simulink library "rotorTemp_lib"  (R2022b)
settings: Solver=VariableStepAuto  StartTime=0.0  StopTime=10.0  RelTol=1e-3
undefined symbols (not defined in the file): raptor_xcp_function
libraries: Raptor_lib x9
settings Model: Creator=serga  LastModifiedBy=serga

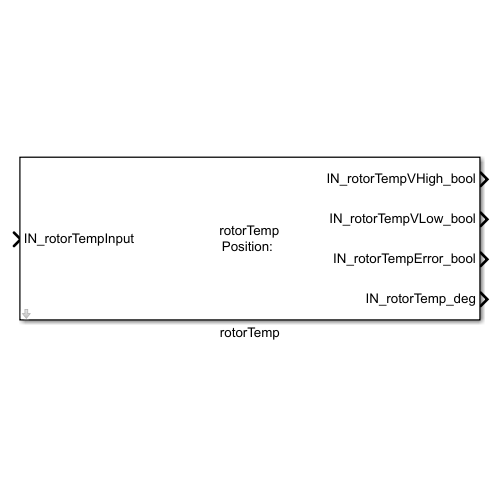
[thumbnail: Simulink's stored preview of the top-level diagram]
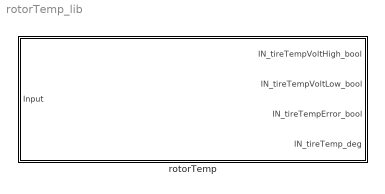
== system rotorTemp_lib ==
  rotorTemp : Subsystem  mask{pos=''}
      mask prompts: pos "Position"
      mask Display:
      | disp(['rotorTemp\n'...
      |     'Position: ' pos]);
      | port_label('input', 1, ['IN_rotorTempInput' pos]);
      | port_label('output', 1, ['IN_rotorTempVHigh' pos '_bool']);
      | port_label('output', 2, ['IN_rotorTempVLow' pos '_bool']);
      | port_label('output', 3, ['IN_rotorTempError' pos '_bool']);
      | port_label('output', 4, ['IN_rotorTemp' pos '_deg']);

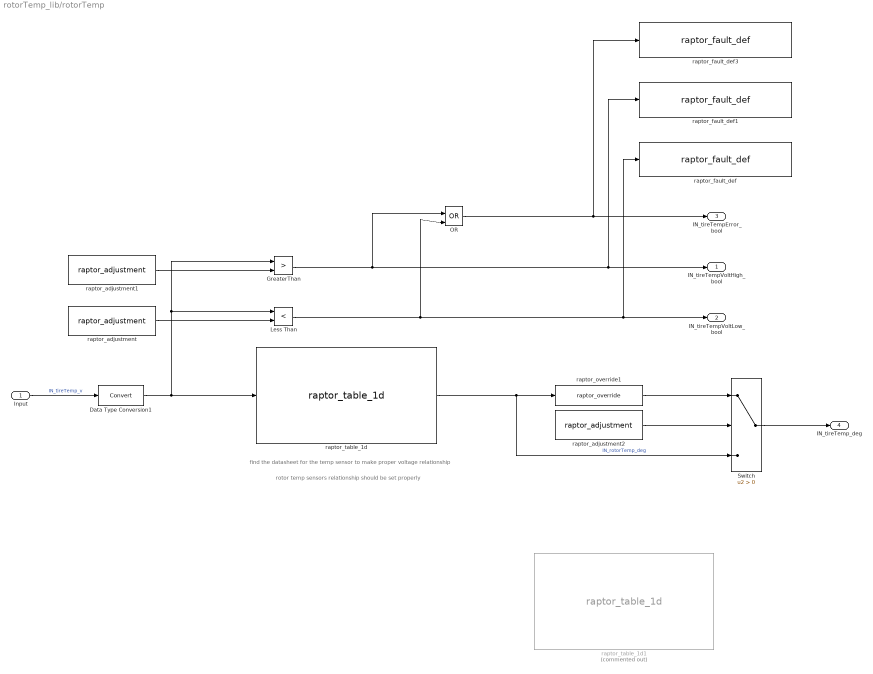
== system rotorTemp_lib/rotorTemp ==
  note: rotor temp sensors relationship should be set properly
  note: find the datasheet for the temp sensor to make proper voltage relationship
  Input : Inport
  Data Type Conversion1 : DataTypeConversion  SaturateOnIntegerOverflow=off  RndMeth=Floor
  GreaterThan : RelationalOperator  Operator=>  OutDataTypeStr=boolean  RndMeth=Simplest  InputSameDT=off
  Less Than : RelationalOperator  Operator=<  OutDataTypeStr=boolean  RndMeth=Simplest  InputSameDT=off
  OR : Logic  Operator=OR  IconShape=distinctive  AllPortsSameDT=off  OutDataTypeStr=boolean
  Switch : Switch  Criteria=u2 > Threshold  SaturateOnIntegerOverflow=off  InputSameDT=off
  raptor_adjustment : Raptor_lib/Data Storage/raptor_adjustment  paramName=['IN_rotorTempLow' pos '_v']  nameSource=Parameter  initValue=0.5  dataType=single  storage=Calibration  calDispType=Number  calEnum={'False', 'True'}  calGain=1.0  calOffset=0.0  calMax=inf  calMin=-inf  calFormat='-1'  calUnit=''  calHelp=''  calAccess=1  calFunction=raptor_xcp_function(gcb)  calDispHeaders=off  calColHeaders={'Col1' 'Col2' 'Col3'}  calRowHeaders={'Row1' 'Row2' 'Row3'}
      settings: SourceProductName=Raptor
  raptor_adjustment1 : Raptor_lib/Data Storage/raptor_adjustment  paramName=['IN_rotorTempHigh' pos '_v']  nameSource=Parameter  initValue=4.5  dataType=single  storage=Calibration  calDispType=Number  calEnum={'False', 'True'}  calGain=1.0  calOffset=0.0  calMax=inf  calMin=-inf  calFormat='-1'  calUnit=''  calHelp=''  calAccess=1  calFunction=raptor_xcp_function(gcb)  calDispHeaders=off  calColHeaders={'Col1' 'Col2' 'Col3'}  calRowHeaders={'Row1' 'Row2' 'Row3'}
      settings: SourceProductName=Raptor
  raptor_adjustment2 : Raptor_lib/Data Storage/raptor_adjustment  paramName=['IN_rotorTemp' pos '_bool']  nameSource=Parameter  initValue=0.00  dataType=boolean  storage=Calibration  calDispType=Number  calEnum={'False', 'True'}  calGain=1.0  calOffset=0.0  calMax=inf  calMin=-inf  calFormat='-1'  calUnit=''  calHelp=''  calAccess=1  calFunction=raptor_xcp_function(gcb)  calDispHeaders=off  calColHeaders={'Col1' 'Col2' 'Col3'}  calRowHeaders={'Row1' 'Row2' 'Row3'}
      settings: SourceProductName=Raptor
  raptor_fault_def : Raptor_lib/Faults/raptor_fault_def  faultName=['IN_rotorTempVLow' pos '_bool']  persist=off  sticky=off  emisRelated=off  singleTrip=off  clearMethod=Standard  xLimit=25  yLimit=50  calEnable=on  addDisable=off  calAccess=1  calFunction='System | FaultManager'
      settings: SourceProductName=Raptor
  raptor_fault_def1 : Raptor_lib/Faults/raptor_fault_def  faultName=['IN_rotorTempVHigh' pos '_bool']  persist=off  sticky=off  emisRelated=off  singleTrip=off  clearMethod=Standard  xLimit=25  yLimit=50  calEnable=on  addDisable=off  calAccess=1  calFunction='System | FaultManager'
      settings: SourceProductName=Raptor
  raptor_fault_def3 : Raptor_lib/Faults/raptor_fault_def  faultName=['IN_rotorTempError' pos '_bool']  persist=off  sticky=off  emisRelated=off  singleTrip=off  clearMethod=Standard  xLimit=25  yLimit=50  calEnable=on  addDisable=off  calAccess=1  calFunction='System | FaultManager'
      settings: SourceProductName=Raptor
  raptor_override1 : Raptor_lib/Data Storage/raptor_override  paramName=['IN_rotorTemp' pos '_deg']  nameSource=Parameter  measurement=Output  calDispType=Number  calEnum={'False', 'True'}  calGain=1.0  calOffset=0.0  calMax=inf  calMin=-inf  calFormat='-1'  calUnit=''  calHelp=''  calAccess=1  calFunction="[raptor_xcp_function(gcb) '|'  'Override']"
      settings: SourceProductName=Raptor
  raptor_table_1d : Raptor_lib/Table Lookup/raptor_table_1d  dataName=['IN_rotorTempVToDeg' pos]  initValue=[0 20 40 60 80 100 120 140 160 180 200 300 400 500 600 700 800]  dataType=double  storage=Calibration  initValueX=[0.5 0.6 0.7 0.8 0.9 1.0 1.1 1.2 1.3 1.4 1.5 2.0 2.5 3.0 3.5 4.0 4.5]  dataTypeXY=double  storageXY=Calibration  calVisible=on  showTable=on  calGain=1.0  calOffset=0.0  calMax=Inf  calMin=-Inf  calFormat='-1'  calUnit='Deg_C'  calHelp=''  showBreakpoint=on  dataNameX=[]  calGainX=1.0  calOffsetX=0.0  calMaxX=Inf  calMinX=-Inf  calFormatX='-1'  calUnitX='V'  calHelpX=''  calAccess=1  calFunction=raptor_xcp_function(gcb)  measureEnable=off  mName=['Data1D_Output']
      settings: SourceProductName=Raptor
  raptor_table_1d1 : Raptor_lib/Table Lookup/raptor_table_1d  Commented=on  dataName=['IN_rotorTempVToDeg' pos]  initValue=[0 20 40 60 80 100 120 140 160 180 200 300 400 500 600 700 800]  dataType=single  storage=Calibration  initValueX=[0.5 0.6 0.7 0.8 0.9 1.0 1.1 1.2 1.3 1.4 1.5 2.0 2.5 3.0 3.5 4.0 4.5]  dataTypeXY=single  storageXY=Calibration  calVisible=on  showTable=on  calGain=1.0  calOffset=0.0  calMax=Inf  calMin=-Inf  calFormat='-1'  calUnit='Deg_C'  calHelp=''  showBreakpoint=on  dataNameX=[]  calGainX=1.0  calOffsetX=0.0  calMaxX=Inf  calMinX=-Inf  calFormatX='-1'  calUnitX='V'  calHelpX=''  calAccess=1  calFunction=raptor_xcp_function(gcb)  measureEnable=off  mName=['Data1D_Output']
      settings: SourceProductName=Raptor
  IN_tireTempVoltHigh_bool : Outport  OutDataTypeStr=boolean
  IN_tireTempVoltLow_bool : Outport  Port=2  OutDataTypeStr=boolean
  IN_tireTempError_bool : Outport  Port=3  OutDataTypeStr=boolean
  IN_tireTemp_deg : Outport  Port=4  OutDataTypeStr=double
  wires:
  Switch/1 -> IN_tireTemp_deg/1
  Less Than/1 -> raptor_fault_def/1, IN_tireTempVoltLow_bool/1, OR/2
  Data Type Conversion1/1 -> GreaterThan/1, Less Than/1, raptor_table_1d/1
  raptor_adjustment1/1 -> GreaterThan/2
  raptor_adjustment/1 -> Less Than/2
  raptor_table_1d/1 -> raptor_override1/1, Switch/3  "IN_rotorTemp_deg"
  raptor_override1/1 -> Switch/1
  OR/1 -> raptor_fault_def3/1, IN_tireTempError_bool/1
  GreaterThan/1 -> OR/1, raptor_fault_def1/1, IN_tireTempVoltHigh_bool/1
  Input/1 -> Data Type Conversion1/1  "IN_tireTemp_v"
  raptor_adjustment2/1 -> Switch/2
